simulink model "Buck_Converter_09102020"  (R2020a)
settings: Solver=VariableStepAuto  StartTime=0.0  StopTime=10.0  RelTol=1e-3
libraries: powerlib x16
settings Model: LastModifiedBy=rajgo

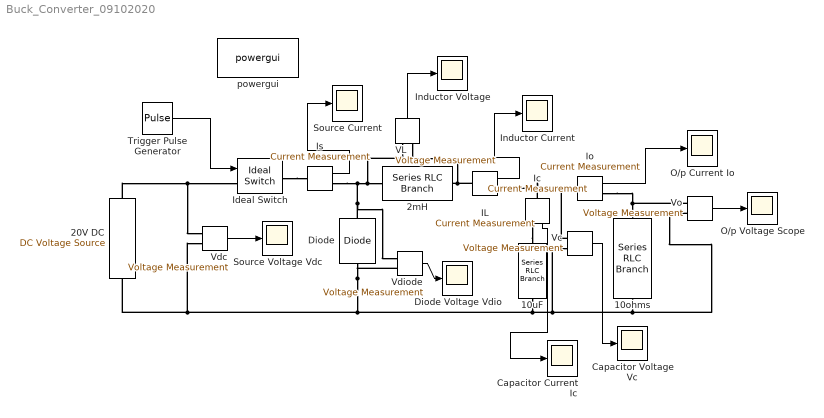
== system Buck_Converter_09102020 ==
  10ohms : powerlib/Elements/Series RLC Branch  LConnTagsString=__new0  RConnTagsString=__new0  BranchType=R  Resistance=10  Inductance=1e-3  SetiL0=off  InitialCurrent=0  Capacitance=1e-6  Setx0=off  InitialVoltage=0  Measurements=None
  10uF : powerlib/Elements/Series RLC Branch  LConnTagsString=__new0  RConnTagsString=__new0  BranchType=C  Resistance=1  Inductance=1e-3  SetiL0=off  InitialCurrent=0  Capacitance=25e-6  Setx0=off  InitialVoltage=0  Measurements=None
  20V DC : powerlib/Electrical Sources/DC Voltage Source  Amplitude=20  Measurements=None
  2mH : powerlib/Elements/Series RLC Branch  LConnTagsString=__new0  RConnTagsString=__new0  BranchType=L  Resistance=1  Inductance=4e-3  SetiL0=off  InitialCurrent=0  Capacitance=1e-6  Setx0=off  InitialVoltage=0  Measurements=None
  Capacitor Current Ic : Scope
  Capacitor Voltage Vc : Scope
  "Diode " : powerlib/Power Electronics/Diode  Ron=0  Lon=0  Vf=0  IC=0  UseSnubber=0  Rs=inf  Cs=0  Measurements=off
  Diode Voltage Vdio : Scope
  IL : powerlib/Measurements/Current Measurement  PhasorSimulation=off  OutputType=Complex  PSBequivalent=0
  Ic : powerlib/Measurements/Current Measurement  PhasorSimulation=off  OutputType=Complex  PSBequivalent=0
  "Ideal Switch " : powerlib/Power Electronics/Ideal Switch  Ron=00.0000000000000000000001  Lon=0  IC=0  Rs=inf  Cs=0  Measurements=off
  Inductor Current : Scope
  Inductor Voltage : Scope
  Io : powerlib/Measurements/Current Measurement  PhasorSimulation=off  OutputType=Complex  PSBequivalent=0
  Is : powerlib/Measurements/Current Measurement  PhasorSimulation=off  OutputType=Complex  PSBequivalent=0
  O/p Current Io : Scope
  O/p Voltage Scope : Scope
  Source Current : Scope
  Source Voltage Vdc : Scope
  Trigger Pulse Generator : DiscretePulseGenerator  PulseType=Time based  Amplitude=20  Period=1/5000  PulseWidth=50
  VL : powerlib/Measurements/Voltage Measurement  PhasorSimulation=off  OutputType=Complex  PSBequivalent=0
  Vc : powerlib/Measurements/Voltage Measurement  PhasorSimulation=off  OutputType=Complex  PSBequivalent=0
  Vdc : powerlib/Measurements/Voltage Measurement  PhasorSimulation=off  OutputType=Complex  PSBequivalent=0
  Vdiode : powerlib/Measurements/Voltage Measurement  PhasorSimulation=off  OutputType=Complex  PSBequivalent=0
  Vo : powerlib/Measurements/Voltage Measurement  PhasorSimulation=off  OutputType=Complex  PSBequivalent=0
  powergui : powerlib/powergui  Priority=1  SimulationMode=Continuous  SampleTime=50e-6  frequency=60  Iterations=50  frequencyindice=0  Pbase=100e6  ErrMax=1e-4  UnitsV=kV  UnitsW=MW  buscounter=0  FunctionMessages=off  echomessages=off  EnableUseOfTLC=off  CurrentSourceSwitches=off  DisableSnubberDevices=off  DisableRonSwitches=off  DisableVfSwitches=off  DisplayEquations=off  AutomaticDiscreteSolvers=off  SolverType=Tustin/Backward Euler (TBE)  Interpol=off  ExternalGateDelay=off  methode=off  Ts=100  x0status=blocks  SPID=on  SwTol=0  HookPort=off  NonlinearTolerance=1e-4  nMaxIteration=100  ContinueOnMaxIteration=off  RestoreLinks=warning  ResistiveCurrentMeasurement=off  Frange=[0:2:500]  Ylog=off  Xlog=on  ShowGrid=off  save=off  variable=ZData  structure=0  ZoomFFT=off  StartTime=0.0  cycles=1  DisplayStyle=1  fundamental=60  FreqAxis=off  MaxFrequency=1000  frequencyindicesteady=1  RmsSteady=1  display=off
  wires:
  Vo/1 -> O/p Voltage Scope/1
  Vdc/1 -> Source Voltage Vdc/1
  VL/1 -> Inductor Voltage/1
  Vdiode/1 -> Diode Voltage Vdio/1
  IL/1 -> Inductor Current/1
  Io/1 -> O/p Current Io/1
  Vc/1 -> Capacitor Voltage Vc/1
  Ic/1 -> Capacitor Current Ic/1
  Is/1 -> Source Current/1
  Trigger Pulse Generator/1 -> "Ideal Switch "/1
  connections:
  20V DC/RConn1 -- Vdc/LConn1 -- "Ideal Switch "/LConn1
  "Diode "/RConn1 -- Vdiode/LConn1 -- VL/LConn1 -- 2mH/LConn1 -- Is/RConn1
  Io/LConn1 -- Ic/LConn1 -- IL/RConn1 -- Vc/LConn1
  10uF/RConn1 -- Vo/LConn2 -- 10ohms/RConn1 -- Vc/LConn2 -- Vdiode/LConn2 -- "Diode "/LConn1 -- Vdc/LConn2 -- 20V DC/LConn1
  IL/LConn1 -- VL/LConn2 -- 2mH/RConn1
  "Ideal Switch "/RConn1 -- Is/LConn1
  Vo/LConn1 -- Io/RConn1 -- 10ohms/LConn1
  Ic/RConn1 -- 10uF/LConn1
